simulink model "Battery_Electrothermal_Model_charge"  (R2017b)
settings: Solver=ode45  StartTime=0.0  StopTime=10.0  RelTol=1e-3  EnableMultiTasking=on
values from neighbouring files (symbols this model uses):
  C12_SOC_c = [397.526659684 455.660832136 435.08783522 460.845064365 457.605812374 417.289828504 416.373906992 359.741413056 321.561704819 1109.14132554 1165.67733205 1135.97600211 ... (72 elements, 9x8)]    [r_rc_rc_scale_cap_A123_26650.mat]
  C12_SOC_d = [187.121968588 287.083505726 346.448009002 395.529439835 387.517274826 389.973134196 432.856765051 486.92921923 512.158935268 425.990733989 614.68708868 771.472592368 ... (72 elements, 9x8)]    [r_rc_rc_scale_cap_A123_26650.mat]
  C22_SOC_c = [8748.48589695 7773.35875681 9404.86567646 8934.73981058 8290.58671366 7592.78422269 7759.44623103 7396.59043829 6151.35152293 16187.7227039 11721.8480541 13157.8579836 ... (72 elements, 9x8)]    [r_rc_rc_scale_cap_A123_26650.mat]
  C22_SOC_d = [2939.81325553 4590.73311898 5504.93546413 5887.5077374 6534.37836712 7765.46899768 10584.7751706 10372.0508438 9238.72693885 5207.86390693 7911.43744944 8879.62137571 ... (72 elements, 9x8)]    [r_rc_rc_scale_cap_A123_26650.mat]
  C_bat = 2.3    [run_model.m]    (also in run_model7459.m = 3.2)
  Cc = 62.7    [run_model.m]    (also in run_model7459.m)
  Cs = 4.5    [run_model.m]    (also in run_model7459.m)
  R12_SOC_c = [0.114339870884 0.105392753268 0.104421193553 0.109821896183 0.114868279838 0.123333154908 0.129174812826 0.149917249373 0.174896487845 0.0420560161846 0.0390948352938 0.0370122837364 ... (72 elements, 9x8)]    [r_rc_rc_scale_cap_A123_26650.mat]
  R12_SOC_d = [0.304806399643 0.213604089624 0.171463520004 0.151183840498 0.140630862434 0.128795299077 0.116857791733 0.112567113582 0.106368362501 0.0943235089866 0.0730697254134 0.0611414736086 ... (72 elements, 9x8)]    [r_rc_rc_scale_cap_A123_26650.mat]
  R22_SOC_c = [0.134518959939 0.17565045702 0.161100627268 0.189032232545 0.205639040497 0.226170473035 0.223651875822 0.181765694192 0.212966950836 0.073628872144 0.0788540822416 0.0792414571734 ... (72 elements, 9x8)]    [r_rc_rc_scale_cap_A123_26650.mat]
  R22_SOC_d = [0.354968099904 0.285293035102 0.286338708953 0.298763853987 0.248762838155 0.178586175471 0.129047399775 0.188406991173 0.174494800676 0.131839238891 0.123225430215 0.132069033134 ... (72 elements, 9x8)]    [r_rc_rc_scale_cap_A123_26650.mat]
  Rc = 1.94    [run_model.m]    (also in run_model7459.m)
  RF = 2    [run_model7459.m]
  Rs2_SOC_c = [0.0771669453735 0.0731809311402 0.0726556782939 0.0729965156794 0.0731758310684 0.0742031005051 0.0721266921026 0.0714211058078 0.0714186176143 0.0374124505155 0.0354566732504 0.0345430657188 ... (72 elements, 9x8)]    [r_rc_rc_scale_cap_A123_26650.mat]
  Rs2_SOC_d = [0.0819458671157 0.0812429476608 0.0803749674507 0.0805513601722 0.0838629023857 0.0850797840015 0.0829875518672 0.0826388888889 0.0812514106148 0.0428124986417 0.0424658903711 0.0428572670451 ... (72 elements, 9x8)]    [r_rc_rc_scale_cap_A123_26650.mat]
  Ru = 15    [run_model.m]    (also in run_model7459.m)
  SOC_0 = 1    [run_model.m]    (also in run_model7459.m = 0.1)
  Tc_0 = 25    [run_model.m]    (also in run_model7459.m)
  Tf = 25    [run_model.m]    (also in run_model7459.m)
  Ts_0 = 25    [run_model.m]    (also in run_model7459.m)
  V_avgC20 = [2.2238 2.29420016335 2.42397187118 2.5176545146 2.57860244484 2.62198160854 2.65395 2.68031425195 2.7033894395 2.72404689537 2.74265 2.75963736975 ... (1001 elements, 1x1001)]    [V_avgC20.mat]
  V_T_stop = 4.2    [run_model7459.m]
undefined symbols (not defined in the file or in its folder): dUdt, SOC_ent
libraries: simulink x1
settings Model: Creator=xinfan  LastModifiedBy=Robert Wygant
settings DataIOCC: LimitDataPoints=on  SaveFormat=Array  SignalLoggingSaveFormat=ModelDataLogs
settings OptimizationCC: ExpressionDepthLimit=2147483647  LifeSpan=inf
settings DebuggingCC: UnderspecifiedInitializationDetection=Classic  MergeDetectMultiDrivingBlocksExec=none  SolverPrmCheckMsg=warning  FcnCallInpInsideContextMsg=warning  StateNameClashWarn=warning  StrictBusMsg=Warning  SFUnexpectedBacktrackingDiag=warning  SFNoUnconditionalDefaultTransitionDiag=warning  SFExecutionAtInitializationDiag=none
settings HardwareCC: ProdBitPerPointer=32  ProdBitPerSizeT=32  ProdBitPerPtrDiffT=32  ProdLargestAtomicFloat=None  ProdIntDivRoundTo=Undefined  ProdEndianess=Unspecified  ProdWordSize=32  ProdHWDeviceType=32-bit Generic
settings ModelReferenceCC: PropagateSignalLabelsOutOfModel=off
settings CodeAppCC: StateflowObjectComments=on
settings GRTTargetCC: TargetLangStandard=C89/C90 (ANSI)  CombineOutputUpdateFcns=off  GRTInterface=on
settings ConfigComp: CovMetricSettings=dw  CovHtmlReporting=on  CovSaveCumulativeToWorkspaceVar=on  CovSaveSingleToWorkspaceVar=on  CovExternalEMLEnable=off

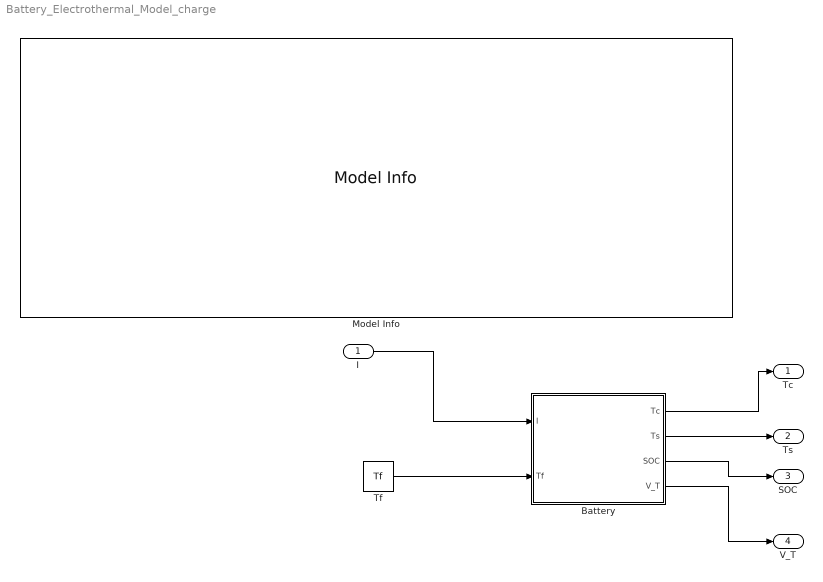
== system Battery_Electrothermal_Model_charge ==
  I : Inport  Interpolate=off
  Battery : Subsystem
  Model Info : simulink/Model-Wide Utilities/Model Info  Frame=on  DisplayStringWithTags=|  HorizontalTextAlignment=Left  LeftAlignmentValue=0.02
      | COPYRIGHT  2013
      | THE REGENTS OF THE UNIVERSITY OF MICHIGAN
      | ALL RIGHTS RESERVED
      | 
      | PERMISSION IS GRANTED TO USE, COPY AND REDISTRIBUTE THIS SOFTWARE FOR NONCOMMERCIAL EDUCATION AND RESEARCH
      | PURPOSES, SO LONG AS NO FEE IS CHARGED, AND SO LONG AS THE COPYRIGHT NOTICE ABOVE, THIS GRANT OF PERMISSION, 
      | AND THE DISCLAIMER BELOW APPEAR IN ALL COPIES MADE; AND SO LONG AS THE NAME OF THE UNIVERSITY OF MICHIGAN IS NOT 
      | USED IN ANY ADVERTISING OR PUBLICITY PERTAINING TO THE USE OR DISTRIBUTION OF THIS SOFTWARE WITHOUT SPECIFIC, 
      | WRITTEN PRIOR AUTHORIZATION.  PERMISSION TO MODIFY OR OTHERWISE CREATE DERIVATIVE WORKS OF THIS SOFTWARE 
      | IS NOT GRANTED.
      | 
      | THIS USE OF THIS SOFTWARE REQUIRES MATLAB(TM) AND SIMULINK(TM), A LICENSED PRODUCT OF THE MATHWORKS, INC. 
      | THE SOFTWARE USER IS SOLELY RESOPNSIBLE FOR OBTAINTING AN APPROPRIATE LICENSE FOR MATLAB(TM) AND SIMULINK(TM).  
      | NO LICENSE TO MATLAB(TM) AND SIMULINK(TM) IS GRANTED, INFERRED OR IMPLIED BY THE DISTRIBUTION OF THIS SOFTWARE.
      | 
      | THIS SOFTWARE IS PROVIDED AS IS, WITHOUT REPRESENTATION AS TO ITS FITNESS FOR ANY PURPOSE, AND WITHOUT WARRANTY 
      | OF ANY KIND, EITHER EXPRESS OR IMPLIED, INCLUDING WITHOUT LIMITATION THE IMPLIED WARRANTIES OF MERCHANTABILITY AND
      | FITNESS FOR A PARTICULAR PURPOSE. THE REGENTS OF THE UNIVERSITY OF MICHIGAN SHALL NOT BE LIABLE FOR ANY DAMAGES,
      | INCLUDING SPECIAL, INDIRECT, INCIDENTAL, OR CONSEQUENTIAL DAMAGES, WITH RESPECT TO ANY CLAIM ARISING OUT OF OR IN
      | CONNECTION WITH THE USE OF THE SOFTWARE, EVEN IF IT HAS BEEN OR IS HEREAFTER ADVISED OF THE POSSIBILITY OF SUCH 
      | DAMAGES.
  Tf : Constant  Value=Tf
  Tc : Outport
  Ts : Outport  Port=2
  SOC : Outport  Port=3
  V_T : Outport  Port=4
  wires:
  Tf/1 -> Battery/2(Tf)
  I/1 -> Battery/1(I)
  Battery/1(Tc) -> Tc/1
  Battery/2(Ts) -> Ts/1
  Battery/3(SOC) -> SOC/1
  Battery/4(V_T) -> V_T/1

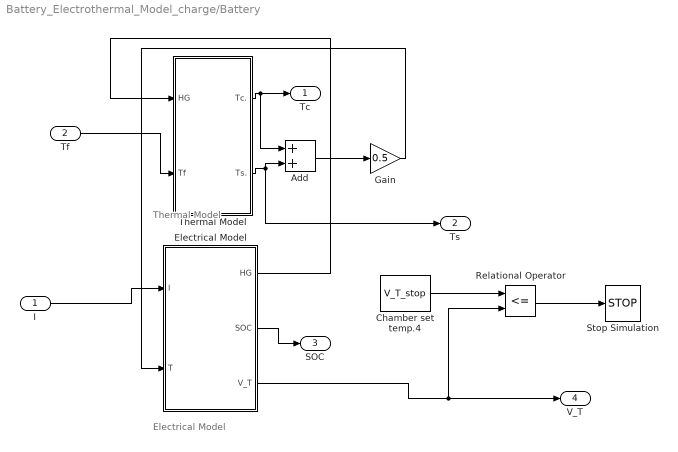
== system Battery_Electrothermal_Model_charge/Battery ==
  note: Electrical Model
  note: Thermal Model
  I : Inport  Interpolate=off
  Tf : Inport  Port=2
  Add : Sum
  Chamber set temp.4 : Constant  Value=V_T_stop
  Electrical Model : Subsystem  Tag=electrical
  Gain : Gain  Gain=0.5
  Relational Operator : RelationalOperator  Operator=<=  OutDataTypeStr=boolean  RndMeth=Simplest
  Stop Simulation : Stop
  Thermal Model : Subsystem
  Tc : Outport
  Ts : Outport  Port=2
  SOC : Outport  Port=3
  V_T : Outport  Port=4
  wires:
  Thermal Model/1(Tc.) -> Add/1, Tc/1
  Electrical Model/1(HG) -> Thermal Model/1(HG)
  Thermal Model/2(Ts.) -> Add/2, Ts/1
  Add/1 -> Gain/1
  Tf/1 -> Thermal Model/2(Tf)
  Gain/1 -> Electrical Model/2(T)
  Relational Operator/1 -> Stop Simulation/1
  Chamber set temp.4/1 -> Relational Operator/1
  I/1 -> Electrical Model/1(I)
  Electrical Model/2(SOC) -> SOC/1
  Electrical Model/3(V_T) -> Relational Operator/2, V_T/1

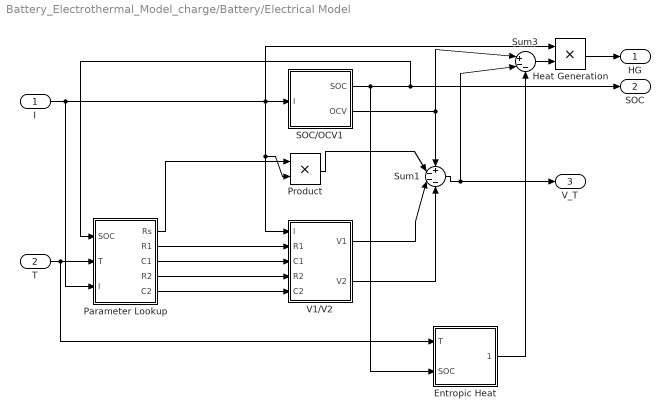
== system Battery_Electrothermal_Model_charge/Battery/Electrical Model ==
  I : Inport
  T : Inport  Port=2
  Entropic Heat : Subsystem
  Heat Generation : Product  RndMeth=Zero
  Parameter Lookup : Subsystem
  Product : Product  RndMeth=Zero
  SOC/OCV1 : Subsystem
  Sum1 : Sum  Inputs=+---
  Sum3 : Sum  Inputs=|+--
  V1/V2 : Subsystem
  HG : Outport
  SOC : Outport  Port=2
  V_T : Outport  Port=3
  wires:
  I/1 -> Parameter Lookup/3(I), Heat Generation/1, Product/2, V1/V2/1(I), SOC/OCV1/1(I)
  V1/V2/1(V1) -> Sum1/3
  Sum1/1 -> V_T/1, Sum3/2
  SOC/OCV1/1(SOC) -> Parameter Lookup/1(SOC), SOC/1, Entropic Heat/2(SOC)
  Product/1 -> Sum1/2
  Sum3/1 -> Heat Generation/2
  SOC/OCV1/2(OCV) -> Sum3/1, Sum1/1
  Parameter Lookup/1(Rs) -> Product/1
  Parameter Lookup/2(R1) -> V1/V2/2(R1)
  Parameter Lookup/4(R2) -> V1/V2/4(R2)
  T/1 -> Parameter Lookup/2(T), Entropic Heat/1(T)
  Heat Generation/1 -> HG/1
  Parameter Lookup/3(C1) -> V1/V2/3(C1)
  Parameter Lookup/5(C2) -> V1/V2/5(C2)
  V1/V2/2(V2) -> Sum1/4
  Entropic Heat/1(HG_ent) -> Sum3/3

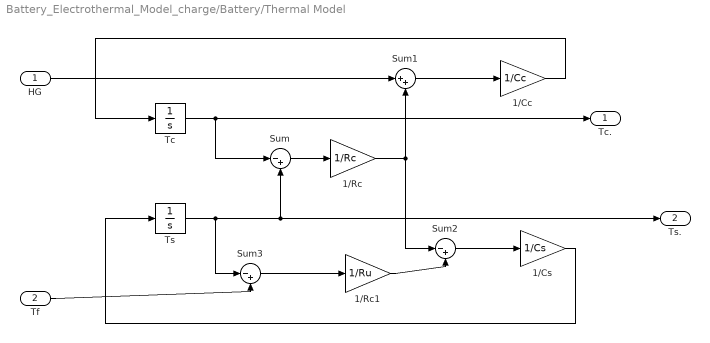
== system Battery_Electrothermal_Model_charge/Battery/Thermal Model ==
  HG : Inport
  Tf : Inport  Port=2
  1/Cc : Gain  Gain=1/Cc
  1/Cs : Gain  Gain=1/Cs
  1/Rc : Gain  Gain=1/Rc
  1/Rc1 : Gain  Gain=1/Ru
  Sum : Sum  Inputs=|-+
  Sum1 : Sum  Inputs=|++
  Sum2 : Sum  Inputs=|-+
  Sum3 : Sum  Inputs=|-+
  Tc : Integrator  InitialCondition=Tc_0
  Ts : Integrator  InitialCondition=Ts_0
  Tc. : Outport
  Ts. : Outport  Port=2
  wires:
  HG/1 -> Sum1/1
  Tf/1 -> Sum3/2
  Ts/1 -> Sum3/1, Sum/2, Ts./1
  Tc/1 -> Sum/1, Tc./1
  Sum/1 -> 1/Rc/1
  1/Rc/1 -> Sum2/1, Sum1/2
  Sum1/1 -> 1/Cc/1
  1/Cc/1 -> Tc/1
  Sum2/1 -> 1/Cs/1
  1/Cs/1 -> Ts/1
  Sum3/1 -> 1/Rc1/1
  1/Rc1/1 -> Sum2/2

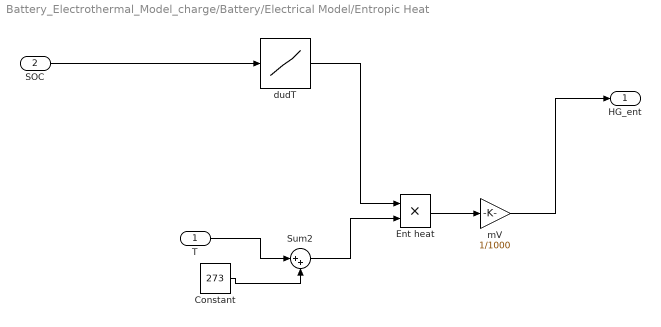
== system Battery_Electrothermal_Model_charge/Battery/Electrical Model/Entropic Heat ==
  T : Inport
  SOC : Inport  Port=2
  Constant : Constant  Value=273
  Ent heat : Product  RndMeth=Zero
  Sum2 : Sum  Inputs=|++
  dudT : Lookup  InputValues=SOC_ent  Table=dUdt
  mV : Gain  Gain=1/1000
  HG_ent : Outport
  wires:
  Sum2/1 -> Ent heat/2
  Constant/1 -> Sum2/2
  T/1 -> Sum2/1
  dudT/1 -> Ent heat/1
  Ent heat/1 -> mV/1
  SOC/1 -> dudT/1
  mV/1 -> HG_ent/1

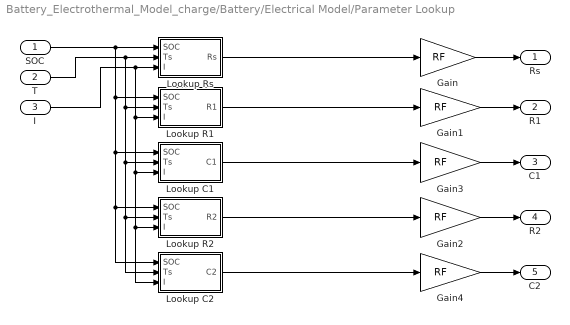
== system Battery_Electrothermal_Model_charge/Battery/Electrical Model/Parameter Lookup ==
  SOC : Inport
  T : Inport  Port=2
  I : Inport  Port=3
  Gain{,1..4} (5 alike) : Gain  Gain=RF
  Lookup C1 : Subsystem
  Lookup C2 : Subsystem
  Lookup R1 : Subsystem
  Lookup R2 : Subsystem
  Lookup Rs : Subsystem
  Rs : Outport
  R1 : Outport  Port=2
  C1 : Outport  Port=3
  R2 : Outport  Port=4
  C2 : Outport  Port=5
  wires:
  SOC/1 -> Lookup Rs/1(SOC), Lookup R1/1(SOC), Lookup C1/1(SOC), Lookup R2/1(SOC), Lookup C2/1(SOC)
  T/1 -> Lookup Rs/2(Ts), Lookup R1/2(Ts), Lookup C1/2(Ts), Lookup R2/2(Ts), Lookup C2/2(Ts)
  I/1 -> Lookup Rs/3(I), Lookup R1/3(I), Lookup C1/3(I), Lookup R2/3(I), Lookup C2/3(I)
  Lookup Rs/1(Rs) -> Gain/1
  Gain3/1 -> C1/1
  Lookup C2/1(C2) -> Gain4/1
  Gain4/1 -> C2/1
  Gain2/1 -> R2/1
  Lookup R2/1(R2) -> Gain2/1
  Gain1/1 -> R1/1
  Gain/1 -> Rs/1
  Lookup R1/1(R1) -> Gain1/1
  Lookup C1/1(C1) -> Gain3/1

== system Battery_Electrothermal_Model_charge/Battery/Electrical Model/SOC//OCV1 ==
  I : Inport
  Avg : Lookup  InputValues=[0:0.001:1]  Table=V_avgC20  LookUpMeth=Interpolation-Use End Values
  Gain1 : Gain  Gain=-1/(3600*C_bat)
  Integrator : Integrator  InitialCondition=SOC_0
  SOC : Outport
  OCV : Outport  Port=2
  wires:
  Integrator/1 -> SOC/1, Avg/1
  Avg/1 -> OCV/1
  I/1 -> Gain1/1
  Gain1/1 -> Integrator/1

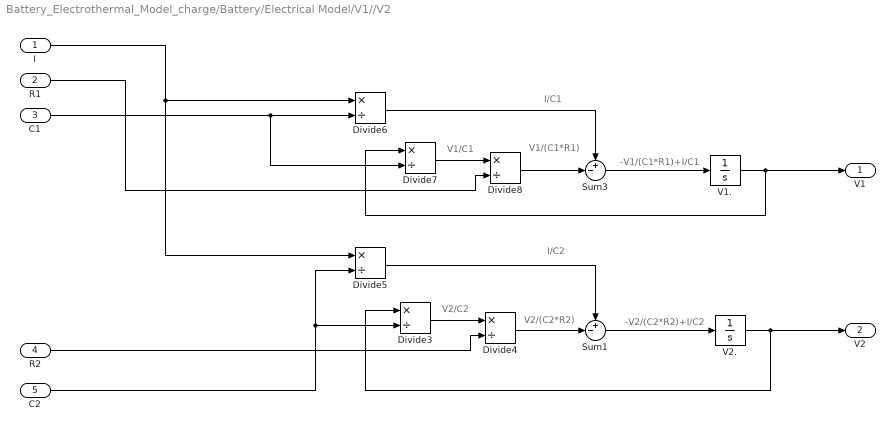
== system Battery_Electrothermal_Model_charge/Battery/Electrical Model/V1//V2 ==
  note: V2/(C2*R2)
  note: -V2/(C2*R2)+I/C2
  note: V2/C2
  note: I/C2
  note: V1/(C1*R1)
  note: I/C1
  note: -V1/(C1*R1)+I/C1
  note: V1/C1
  I : Inport
  R1 : Inport  Port=2
  C1 : Inport  Port=3
  R2 : Inport  Port=4
  C2 : Inport  Port=5
  Divide{3..8} (6 alike) : Product  Inputs=*/  RndMeth=Zero
  Sum1 : Sum  Inputs=+-|
  Sum3 : Sum  Inputs=+-|
  V1. : Integrator
  V2. : Integrator
  V1 : Outport
  V2 : Outport  Port=2
  wires:
  C1/1 -> Divide6/2, Divide7/2
  V2./1 -> Divide3/1, V2/1
  Divide4/1 -> Sum1/2
  Sum1/1 -> V2./1
  C2/1 -> Divide5/2, Divide3/2
  Divide3/1 -> Divide4/1
  R2/1 -> Divide4/2
  Divide5/1 -> Sum1/1
  V1./1 -> Divide7/1, V1/1
  Divide8/1 -> Sum3/2
  Sum3/1 -> V1./1
  Divide6/1 -> Sum3/1
  Divide7/1 -> Divide8/1
  I/1 -> Divide5/1, Divide6/1
  R1/1 -> Divide8/2

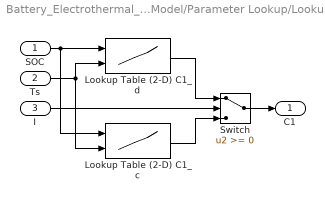
== system Battery_Electrothermal_Model_charge/Battery/Electrical Model/Parameter Lookup/Lookup C1 ==
  SOC : Inport
  Ts : Inport  Port=2
  I : Inport  Port=3
  Lookup Table (2-D) C1_c : Lookup2D  RowIndex=SOC_Temp_c  ColumnIndex=Temp  Table=C12_SOC_c
  Lookup Table (2-D) C1_d : Lookup2D  RowIndex=SOC_Temp_d  ColumnIndex=Temp  Table=C12_SOC_d
  Switch : Switch
  C1 : Outport
  wires:
  Ts/1 -> Lookup Table (2-D) C1_c/2, Lookup Table (2-D) C1_d/2
  SOC/1 -> Lookup Table (2-D) C1_c/1, Lookup Table (2-D) C1_d/1
  Lookup Table (2-D) C1_c/1 -> Switch/3
  Lookup Table (2-D) C1_d/1 -> Switch/1
  Switch/1 -> C1/1
  I/1 -> Switch/2

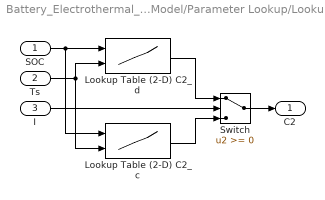
== system Battery_Electrothermal_Model_charge/Battery/Electrical Model/Parameter Lookup/Lookup C2 ==
  SOC : Inport
  Ts : Inport  Port=2
  I : Inport  Port=3
  Lookup Table (2-D) C2_c : Lookup2D  RowIndex=SOC_Temp_c  ColumnIndex=Temp  Table=C22_SOC_c  LookUpMeth=Interpolation-Use End Values
  Lookup Table (2-D) C2_d : Lookup2D  RowIndex=SOC_Temp_d  ColumnIndex=Temp  Table=C22_SOC_d  LookUpMeth=Interpolation-Use End Values
  Switch : Switch
  C2 : Outport
  wires:
  Switch/1 -> C2/1
  Lookup Table (2-D) C2_d/1 -> Switch/1
  Lookup Table (2-D) C2_c/1 -> Switch/3
  SOC/1 -> Lookup Table (2-D) C2_c/1, Lookup Table (2-D) C2_d/1
  Ts/1 -> Lookup Table (2-D) C2_c/2, Lookup Table (2-D) C2_d/2
  I/1 -> Switch/2

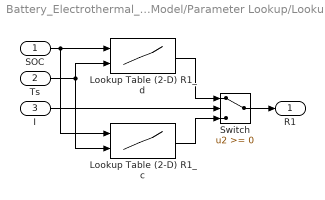
== system Battery_Electrothermal_Model_charge/Battery/Electrical Model/Parameter Lookup/Lookup R1 ==
  SOC : Inport
  Ts : Inport  Port=2
  I : Inport  Port=3
  Lookup Table (2-D) R1_c : Lookup2D  RowIndex=SOC_Temp_c  ColumnIndex=Temp  Table=R12_SOC_c
  Lookup Table (2-D) R1_d : Lookup2D  RowIndex=SOC_Temp_d  ColumnIndex=Temp  Table=R12_SOC_d
  Switch : Switch
  R1 : Outport
  wires:
  Ts/1 -> Lookup Table (2-D) R1_d/2, Lookup Table (2-D) R1_c/2
  SOC/1 -> Lookup Table (2-D) R1_d/1, Lookup Table (2-D) R1_c/1
  Lookup Table (2-D) R1_c/1 -> Switch/3
  Lookup Table (2-D) R1_d/1 -> Switch/1
  I/1 -> Switch/2
  Switch/1 -> R1/1

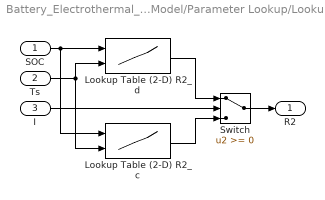
== system Battery_Electrothermal_Model_charge/Battery/Electrical Model/Parameter Lookup/Lookup R2 ==
  SOC : Inport
  Ts : Inport  Port=2
  I : Inport  Port=3
  Lookup Table (2-D) R2_c : Lookup2D  RowIndex=SOC_Temp_c  ColumnIndex=Temp  Table=R22_SOC_c  LookUpMeth=Interpolation-Use End Values
  Lookup Table (2-D) R2_d : Lookup2D  RowIndex=SOC_Temp_d  ColumnIndex=Temp  Table=R22_SOC_d  LookUpMeth=Interpolation-Use End Values
  Switch : Switch
  R2 : Outport
  wires:
  Switch/1 -> R2/1
  I/1 -> Switch/2
  Lookup Table (2-D) R2_d/1 -> Switch/1
  Lookup Table (2-D) R2_c/1 -> Switch/3
  SOC/1 -> Lookup Table (2-D) R2_d/1, Lookup Table (2-D) R2_c/1
  Ts/1 -> Lookup Table (2-D) R2_d/2, Lookup Table (2-D) R2_c/2

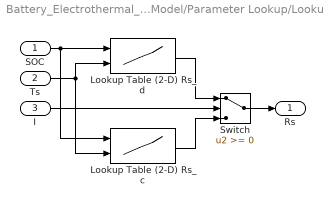
== system Battery_Electrothermal_Model_charge/Battery/Electrical Model/Parameter Lookup/Lookup Rs ==
  SOC : Inport
  Ts : Inport  Port=2
  I : Inport  Port=3
  Lookup Table (2-D) Rs_c : Lookup2D  RowIndex=SOC_Temp_c  ColumnIndex=Temp  Table=Rs2_SOC_c
  Lookup Table (2-D) Rs_d : Lookup2D  RowIndex=SOC_Temp_d  ColumnIndex=Temp  Table=Rs2_SOC_d
  Switch : Switch
  Rs : Outport
  wires:
  Switch/1 -> Rs/1
  I/1 -> Switch/2
  Lookup Table (2-D) Rs_d/1 -> Switch/1
  Lookup Table (2-D) Rs_c/1 -> Switch/3
  SOC/1 -> Lookup Table (2-D) Rs_d/1, Lookup Table (2-D) Rs_c/1
  Ts/1 -> Lookup Table (2-D) Rs_d/2, Lookup Table (2-D) Rs_c/2
